simulink library "me375_robot"  (R2023a)
settings: Solver=VariableStepAuto  StartTime=0.0  StopTime=10.0  RelTol=1e-3
libraries: arduinolib x18, simulink x10, arduinosensorlib x2, $bdroot x1
settings Model: Creator=siche  LastModifiedBy=Zamira

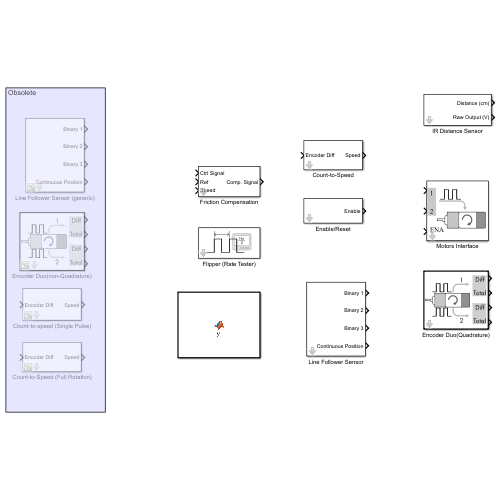
[thumbnail: Simulink's stored preview of the top-level diagram]
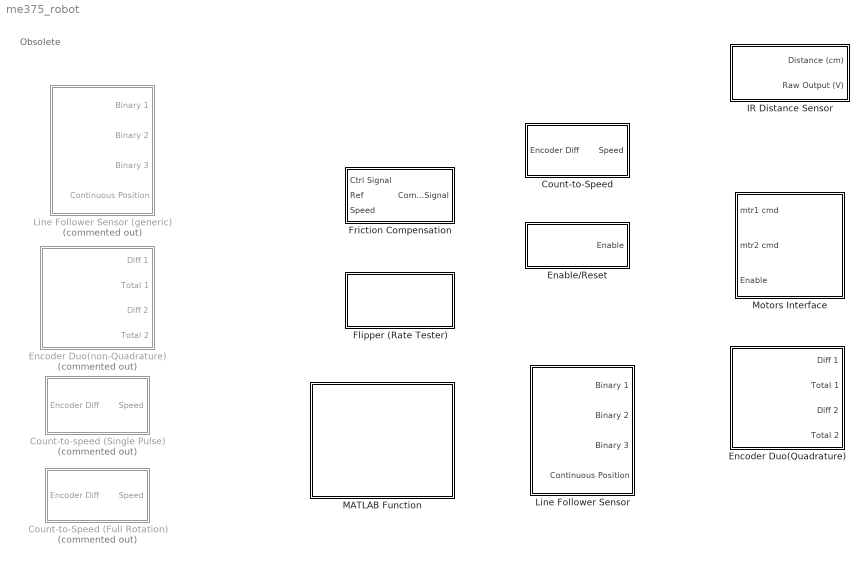
== system me375_robot ==
  note: Obsolete
  Count-to-Speed : Subsystem  mask{cpr=8, Value=184, stop_timeout=15}
      mask prompts: cpr "Window Width"; Value "Count per Wheel Revolution"; stop_timeout "Stop Timeout"
      mask TypeOptions cpr: Pulse Counter/Wrap To Zero/Threshold | Pulse Counter/Constant4/Value | Pulse Counter/Switch/Threshold | Pulse Counter/Switch2/Threshold | Pulse Timing/Constant1/Value
      mask TypeOptions Value: cpr_wheel/Value
      mask TypeOptions stop_timeout: Stop Detection/Wrap To Zero/Threshold | Stop Detection/Switch2/Threshold
      mask DialogControl DescGroupVar Prompt: Encoder Readout Processing
      mask DialogControl DescTextVar Prompt: This block estimates the speed based on the time taken for the encoder to report certain number of counts, specified below as window width. It also accounts for the reduction by the gearbox.
      mask DialogControl Control2 Prompt: This parameter controls the amount of incoming pulses used to estimate the speed. A value too small results in loss in accuracy for high speed, while an overly large value leads to delay at low speeds.
      mask DialogControl Control3 Prompt: The block determines the motor has stopped after recieving this number of consecutive counts of zero.
  Count-to-Speed (Full Rotation) : Subsystem  Commented=on  mask{Value=46, cpr=12, stop_timeout=15}
      mask prompts: Value "Count per Wheel Revolution"; cpr "Count per Rotor Revolution"; stop_timeout "Stop Timeout"
      mask TypeOptions Value: cpr_wheel/Value
      mask TypeOptions cpr: Pulse Counter/Wrap To Zero/Threshold | Pulse Counter/Constant4/Value | Pulse Counter/Switch/Threshold | Pulse Counter/Switch2/Threshold | Pulse Timing/Constant1/Value
      mask TypeOptions stop_timeout: Stop Detection/Wrap To Zero/Threshold | Stop Detection/Switch2/Threshold
      mask DialogControl DescGroupVar Prompt: Encoder Readout Processing
      mask DialogControl DescTextVar Prompt: This block estimates the speed of a motor from the number of encoder pulses recieved since the last iteration of the control loop
      mask DialogControl Control2 Prompt: Encoder count per revolution of the rotor before gearbox. Use 3 for non-quadrature encoder, 12 for quadrature encoder
      mask DialogControl Control3 Prompt: The block determines the motor has stopped after recieving this number of consecutive counts of zero.
  Count-to-speed (Single Pulse) : Subsystem  Commented=on  mask{Value=46, Threshold=15}
      mask prompts: Value "Count per Revolution"; Threshold "Stopping Timeout"
      mask TypeOptions Value: cpr/Value
      mask TypeOptions Threshold: Stop Detection/Wrap To Zero/Threshold
      mask DialogControl DescGroupVar Prompt: Wheel Speed Calculation from Encoder Output
      mask DialogControl DescTextVar Prompt: This block estimates the speed of a motor from the number of encoder pulses recieved since the last iteration of the control loop.
      mask DialogControl Control2 Prompt: Note: This block assumes no more than one incoming encoder count per iteration. If more than one encoder count is expected, one should utilize the Count-to-Speed(Full Rotation) block to avoid exceeding the range of measurement.
      mask DialogControl Control4 Prompt: Count per Revolution = (encoder count per revolution of the motor) x (gear ratio)
      mask DialogControl Control3 Prompt: The block determines the motor has stopped after recieving this number of consecutive counts of zero.
  Enable/Reset : Subsystem  mask{PinEnable=20, enable_override=off}
      mask prompts: PinEnable "Pin number"; enable_override "Button Override"
      mask TypeOptions PinEnable: External Interrupt/Pin
      mask DialogControl DescGroupVar Prompt: Enable/Rest
      mask DialogControl DescTextVar Prompt: Waits for a specified pin to go HIGH before sending out a HIGH as well. This allows one to use external hardware, like a button, to "enable" the connecting block to start functioning.
      mask DialogControl Control2 Prompt: If checked, the robot will start running right after the simulation starts instead of waiting for the button to be pressed.
  Encoder Duo(Quadrature) : Subsystem  TreatAsAtomicUnit=on  mask{mtr_2_dir=on, InputA_enc2=18, InputB_enc2=19, mtr_1_dir=off, InputA_enc1=3, InputB_enc1=2}
      mask prompts: mtr_2_dir "Reverse"; InputA_enc2 "Input A:"; InputB_enc2 "Input B:"; mtr_1_dir "Reverse"; InputA_enc1 "Input A:"; InputB_enc1 "Input B:"
      mask TypeOptions InputA_enc2: Encoder1/InputA
      mask TypeOptions InputB_enc2: Encoder1/InputB
      mask TypeOptions InputA_enc1: Encoder/InputA
      mask TypeOptions InputB_enc1: Encoder/InputB
      mask DialogControl DescTextVar Prompt: Interface with an encoder when only one external interrupt pin is available on the Arduino side. Resolution is 3 counts per revolution of the rotor.
      mask DialogControl ParameterGroupVar Prompt: Pin Settings
      mask DialogControl Container4 Prompt: Motor 1
      mask DialogControl Container5 Prompt: Motor 2
      mask Display: image('encoder_img.svg');
  Encoder Duo(non-Quadrature) : Subsystem  Commented=on  TreatAsAtomicUnit=on  mask{mtr_1_dir=off, pin_intr_1=2, pin_non_intr_1=4, mtr_2_dir=on, pin_intr_2=3, pin_non_intr_2=5, intr_pulledUp_1=on, non_intr_pulledUp_2=Input Pullup, intr_pulledUp_2=on, non_intr_pulledUp_1=Input Pullup, isInputPullup=on}
      mask prompts: mtr_1_dir "Reverse"; pin_intr_1 "Interrupt Pin"; pin_non_intr_1 "Non-interrupt Pin"; mtr_2_dir "Reverse"; pin_intr_2 "Interrupt Pin"; pin_non_intr_2 "Non-interrupt Pin"; intr_pulledUp_1 "Pull-Up Input Pin"; non_intr_pulledUp_2 "Pin mode:"; intr_pulledUp_2 "Pull-Up Input Pin"; non_intr_pulledUp_1 "Pin mode:"; isInputPullup "Pull up"
      mask TypeOptions pin_intr_1: External Interrupt/Pin
      mask TypeOptions pin_non_intr_1:
      | Function-Call
      | Subsystem/Digital Input1/pinNumber
      mask TypeOptions pin_intr_2: External Interrupt1/Pin
      mask TypeOptions pin_non_intr_2:
      | Function-Call
      | Subsystem1/Digital Input1/pinNumber
      mask TypeOptions intr_pulledUp_1: External Interrupt/PullUp
      mask TypeOptions non_intr_pulledUp_2:
      | Function-Call
      | Subsystem1/Digital Input1/mode
      mask TypeOptions intr_pulledUp_2: External Interrupt1/PullUp
      mask TypeOptions non_intr_pulledUp_1:
      | Function-Call
      | Subsystem/Digital Input1/mode
      mask DialogControl DescTextVar Prompt: Interface with an encoder when only one external interrupt pin is available on the Arduino side. Resolution is 3 counts per revolution of the rotor.
      mask DialogControl ParameterGroupVar Prompt: Pin Settings
      mask DialogControl Container4 Prompt: Motor 1
      mask DialogControl Container5 Prompt: Motor 2
      mask DialogControl Container3 Prompt: Pull Up Input
      mask DialogControl Control2 Prompt: The encoders on the Skitter robot require pull-up resistors. Uncheck this box if the resistors are available from the driver board.
      mask Display: image('encoder_img.svg');
  Flipper (Rate Tester) : Subsystem  mask{pinNumber=37}
      mask prompts: pinNumber "Pin number:"
      mask TypeOptions pinNumber: Digital Output/pinNumber
      mask DialogControl DescGroupVar Prompt: Pin State "Flipper"
      mask DialogControl DescTextVar Prompt: For loop rate testing. Use a frequency measurement device (e.g., oscilliscope or multimeter) across the set pin and GND. The frequency at which the control loop runs is twice the measured frequency.
      mask Display: image('flipper_img.svg',[12 8 80 40]);
  Friction Compensation : Subsystem  mask{fric_val=0}
      mask prompts: fric_val "Deadband"
      mask TypeOptions fric_val: Constant1/Value
      mask DialogControl Control2 Prompt: Put the deadband value below to compensate for it:
  IR Distance Sensor : Subsystem  mask{pinNumber=0, CalibValsEnabled=off, Gain4=-4.3019, Gain5=239.1904, Gain6=-0.6848, Gain7=48.1191}
      mask prompts: pinNumber "Pin Number: A"; CalibValsEnabled "Enable Editing"; Gain4 "a1"; Gain5 "k1"; Gain6 "a2"; Gain7 "k2"
      mask TypeOptions pinNumber: Analog Input/pinNumber
      mask TypeOptions Gain4: Gain4/Gain
      mask TypeOptions Gain5: Gain5/Gain
      mask TypeOptions Gain6: Gain6/Gain
      mask TypeOptions Gain7: Gain7/Gain
      mask DialogControl DescTextVar Prompt: This block reads output from a SHARP GP2Y0A21YK0F infrared distance sensor via a 5V/10bit analog input pin.
      mask DialogControl Container4 Prompt: Pin
      mask DialogControl Control2 Prompt: Select analog input pin for the sensor.
      mask DialogControl Container5 Prompt: Calibration
      mask DialogControl Control3 Prompt: The voltage output (u) of the sensor is converted to distance in centimeters (D) by the sum of two exponential functions:
  Line Follower Sensor : Subsystem  mask{Value=650, cont_thresh=256}
      mask prompts: Value "Binary Threshold"; cont_thresh "Continuous Position Correction Threshold"
      mask TypeOptions Value: bin_threshold/Value
      mask TypeOptions cont_thresh: Averaging/Constant/Value | Averaging/Constant1/Value | Averaging/Switch/Threshold | Averaging/Switch1/Threshold
      mask DialogControl Container2 Prompt: Line Follower
      mask DialogControl Control3 Prompt: Uses the three light sensors to determine where the line is likely to be.
      mask DialogControl ParameterGroupVar Prompt: Parameter
      mask DialogControl Control2 Prompt: The Binary Threshold sets the cutoff for the sensors' raw readings, which range from 0 to 1024, before it outputs that it has detected something.
  Line Follower Sensor (generic) : Subsystem  Commented=on  mask{Value=650}
      mask prompts: Value "Binary Threshold"
      mask TypeOptions Value: bin_threshold/Value
      mask DialogControl Container2 Prompt: Line Follower
      mask DialogControl Control3 Prompt: Uses the three light sensors to determine where the line is likely to be.
      mask DialogControl ParameterGroupVar Prompt: Parameter
      mask DialogControl Control2 Prompt: The Binary Threshold sets the cutoff for the sensors' raw readings, which range from 0 to 1024, before it outputs that it has detected something.
  MATLAB Function : MATLAB Function  TreatAsAtomicUnit=on
  Motors Interface : Subsystem  mask{Value=1, pinNumber0=6, pinNumber2=7, pinNumber1=8, pinNumber3=9, desiredFrequency=31372.55}
      mask prompts: Value "u="; pinNumber0 "Out 1"; pinNumber2 "Out 2"; pinNumber1 "Out 1"; pinNumber3 "Out 2"; desiredFrequency "Desired:"
      mask TypeOptions Value: max_input_scaling/Value
      mask TypeOptions pinNumber0: PWM/pinNumber
      mask TypeOptions pinNumber2: PWM2/pinNumber
      mask TypeOptions pinNumber1: PWM1/pinNumber
      mask TypeOptions pinNumber3: PWM3/pinNumber
      mask TypeOptions desiredFrequency: PWM/desiredFrequency | PWM1/desiredFrequency | PWM2/desiredFrequency | PWM3/desiredFrequency
      mask DialogControl DescGroupVar Prompt: PWM Speed Control Interface
      mask DialogControl DescTextVar Prompt: This block converts a control signal to a PWM signal with appropriate duty cycle.
      mask DialogControl Container5 Prompt: Control Signal Range
      mask DialogControl Control2 Prompt: The input control signal should have a value between [-u, u]
      mask DialogControl ParameterGroupVar Prompt: Output Pin Settings
      mask DialogControl Container3 Prompt: Motor 1
      mask DialogControl Container4 Prompt: Motor 2
      mask DialogControl Container7 Prompt: PWM Frequency
      mask Display: image('motor_interface_img.svg');

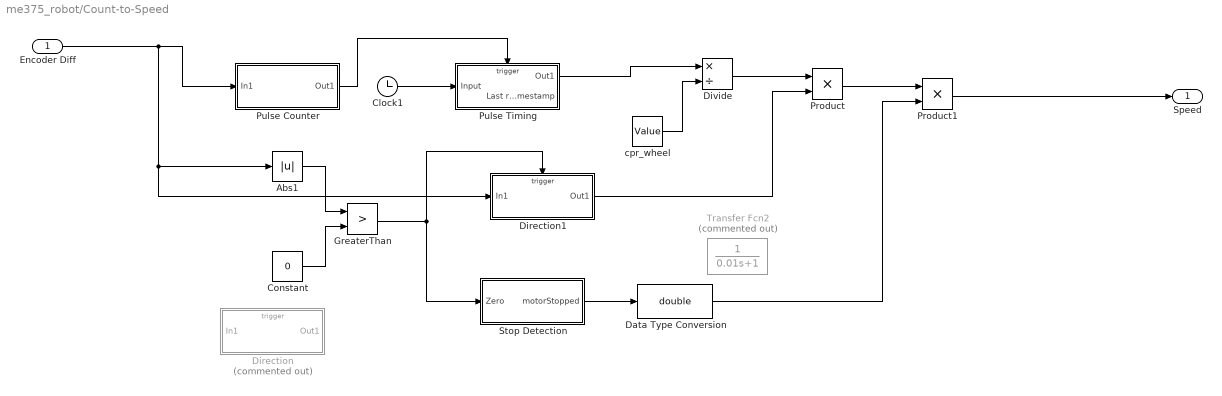
== system me375_robot/Count-to-Speed ==
  Encoder Diff : Inport
  Abs1 : Abs  SaturateOnIntegerOverflow=off
  Clock1 : Clock
  Constant : Constant  Value=0
  Data Type Conversion : DataTypeConversion  OutDataTypeStr=double  SaturateOnIntegerOverflow=off  RndMeth=Floor
  Direction : Subsystem  Commented=on  TreatAsAtomicUnit=on
  Direction1 : Subsystem  TreatAsAtomicUnit=on
  Divide : Product  Inputs=*/
  GreaterThan : RelationalOperator  Operator=>  OutDataTypeStr=boolean  RndMeth=Simplest  InputSameDT=off
  Product : Product
  Product1 : Product
  Pulse Counter : Subsystem
  Pulse Timing : Subsystem  TreatAsAtomicUnit=on
  Stop Detection : Subsystem
  Transfer Fcn2 : TransferFcn  Commented=on  Denominator=[0.01 1]
  cpr_wheel : Constant  Value=Value
  Speed : Outport
  wires:
  Product1/1 -> Speed/1
  cpr_wheel/1 -> Divide/2
  Product/1 -> Product1/1
  Divide/1 -> Product/1
  Abs1/1 -> GreaterThan/1
  Clock1/1 -> Pulse Timing/1(Input)
  Pulse Timing/1(Out1) -> Divide/1
  Constant/1 -> GreaterThan/2
  Pulse Counter/1(Out1) -> Pulse Timing/Trigger
  Encoder Diff/1 -> Pulse Counter/1(In1), Abs1/1, Direction1/1(In1)
  GreaterThan/1 -> Stop Detection/1(Zero), Direction1/Trigger
  Direction1/1(Out1) -> Product/2
  Data Type Conversion/1 -> Product1/2
  Stop Detection/1(motorStopped) -> Data Type Conversion/1

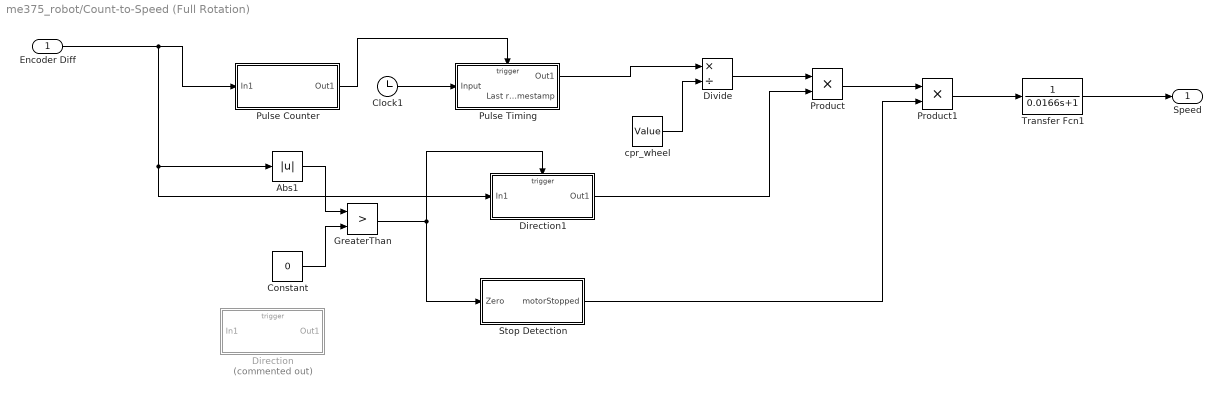
== system me375_robot/Count-to-Speed (Full Rotation) ==
  Encoder Diff : Inport
  Abs1 : Abs  SaturateOnIntegerOverflow=off
  Clock1 : Clock
  Constant : Constant  Value=0
  Direction : Subsystem  Commented=on  TreatAsAtomicUnit=on
  Direction1 : Subsystem  TreatAsAtomicUnit=on
  Divide : Product  Inputs=*/
  GreaterThan : RelationalOperator  Operator=>  OutDataTypeStr=boolean  RndMeth=Simplest  InputSameDT=off
  Product : Product
  Product1 : Product
  Pulse Counter : Subsystem
  Pulse Timing : Subsystem  TreatAsAtomicUnit=on
  Stop Detection : Subsystem
  Transfer Fcn1 : TransferFcn  Denominator=[0.0166 1]
  cpr_wheel : Constant  Value=Value
  Speed : Outport
  wires:
  GreaterThan/1 -> Direction1/Trigger, Stop Detection/1(Zero)
  Encoder Diff/1 -> Direction1/1(In1), Abs1/1, Pulse Counter/1(In1)
  Pulse Counter/1(Out1) -> Pulse Timing/Trigger
  Constant/1 -> GreaterThan/2
  Pulse Timing/1(Out1) -> Divide/1
  Clock1/1 -> Pulse Timing/1(Input)
  Abs1/1 -> GreaterThan/1
  Divide/1 -> Product/1
  Direction1/1(Out1) -> Product/2
  Product/1 -> Product1/1
  Stop Detection/1(motorStopped) -> Product1/2
  cpr_wheel/1 -> Divide/2
  Product1/1 -> Transfer Fcn1/1
  Transfer Fcn1/1 -> Speed/1

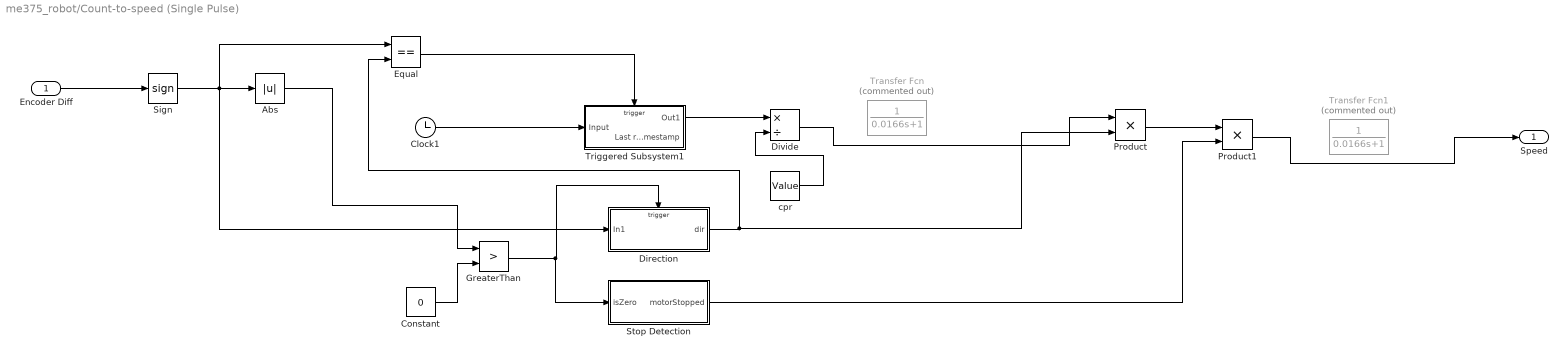
== system me375_robot/Count-to-speed (Single Pulse) ==
  Encoder Diff : Inport
  Abs : Abs  SaturateOnIntegerOverflow=off
  Clock1 : Clock
  Constant : Constant  Value=0
  Direction : Subsystem  TreatAsAtomicUnit=on
  Divide : Product  Inputs=*/
  Equal : RelationalOperator  Operator===  OutDataTypeStr=boolean  RndMeth=Simplest  InputSameDT=off
  GreaterThan : RelationalOperator  Operator=>  OutDataTypeStr=boolean  RndMeth=Simplest  InputSameDT=off
  Product : Product
  Product1 : Product
  Sign : Signum
  Stop Detection : Subsystem
  Transfer Fcn : TransferFcn  Commented=on  Denominator=[0.0166 1]
  Transfer Fcn1 : TransferFcn  Commented=on  Denominator=[0.0166 1]
  Triggered Subsystem1 : Subsystem  TreatAsAtomicUnit=on
  cpr : Constant  Value=Value
  Speed : Outport
  wires:
  GreaterThan/1 -> Stop Detection/1(isZero), Direction/Trigger
  Constant/1 -> GreaterThan/2
  Triggered Subsystem1/1(Out1) -> Divide/1
  Clock1/1 -> Triggered Subsystem1/1(Input)
  Abs/1 -> GreaterThan/1
  Direction/1(dir) -> Product/2, Equal/2
  Product/1 -> Product1/1
  Stop Detection/1(motorStopped) -> Product1/2
  Encoder Diff/1 -> Sign/1
  Sign/1 -> Equal/1, Direction/1(In1), Abs/1
  Equal/1 -> Triggered Subsystem1/Trigger
  cpr/1 -> Divide/2
  Product1/1 -> Speed/1
  Divide/1 -> Product/1

== system me375_robot/Enable//Reset ==
  Constant : Constant  Value=enable_override
  Cool Down : TransferFcn  Denominator=[0.1 1]
  Data Type Conversion : DataTypeConversion  SaturateOnIntegerOverflow=off  RndMeth=Floor
  Data Type Conversion1 : DataTypeConversion  OutDataTypeStr=double  SaturateOnIntegerOverflow=off  RndMeth=Floor
  Digital Input : arduinolib/Digital Input  pinNumber=5  mode=Input Pullup  Direction=input  SampleTime=0.02  blockPlatform=arduino
  External Interrupt : arduinolib/External Interrupt  Pin=PinEnable  PullUp=on  Mode=FALLING  InterruptSimulationInput=off
  OR : Logic  Operator=OR  IconShape=distinctive  AllPortsSameDT=off  OutDataTypeStr=boolean
  RT : RateTransition  Deterministic=off  OutPortSampleTime=0.002
  RT1 : RateTransition  Deterministic=off
  Subsystem : Subsystem
  Enable : Outport
  wires:
  RT/1 -> Data Type Conversion/1
  Subsystem/1(Enable Out) -> RT/1
  RT1/1 -> Subsystem/1(Cool Down Signal)
  Data Type Conversion/1 -> OR/2, Cool Down/1
  Cool Down/1 -> RT1/1
  Constant/1 -> OR/1
  OR/1 -> Data Type Conversion1/1
  Data Type Conversion1/1 -> Enable/1
  Digital Input/1 -> Subsystem/Trigger

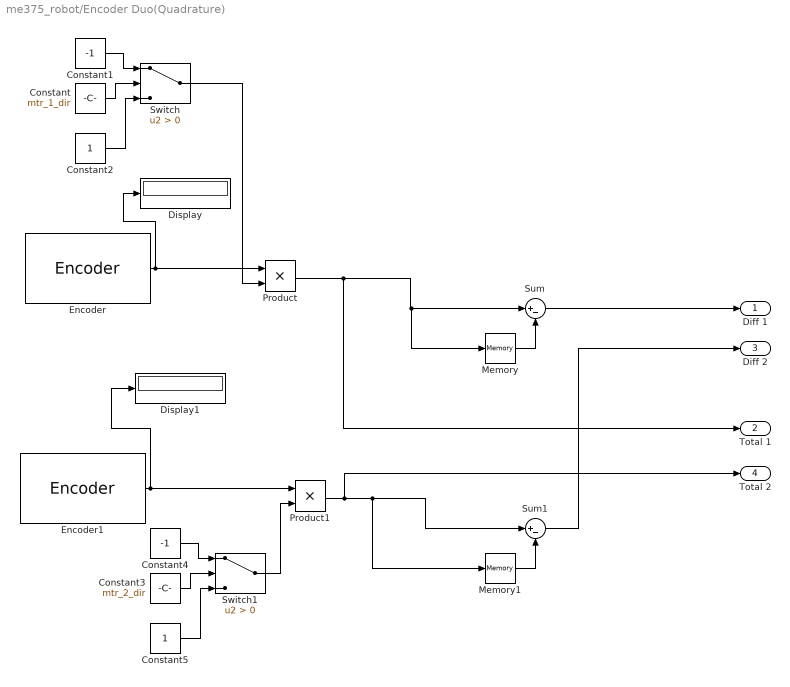
== system me375_robot/Encoder Duo(Quadrature) ==
  Constant : Constant  Value=mtr_1_dir
  Constant1 : Constant  Value=-1
  Constant2 : Constant
  Constant3 : Constant  Value=mtr_2_dir
  Constant4 : Constant  Value=-1
  Constant5 : Constant
  Display : Display
  Display1 : Display
  Encoder : arduinosensorlib/Encoder  InputA=InputA_enc1  InputB=InputB_enc1  Mode=No reset  SampleTime=-1
  Encoder1 : arduinosensorlib/Encoder  InputA=InputA_enc2  InputB=InputB_enc2  Mode=No reset  SampleTime=-1
  Memory : Memory
  Memory1 : Memory
  Product : Product
  Product1 : Product
  Sum : Sum  Inputs=|+-
  Sum1 : Sum  Inputs=|+-
  Switch : Switch  Criteria=u2 > Threshold  SaturateOnIntegerOverflow=off  InputSameDT=off
  Switch1 : Switch  Criteria=u2 > Threshold  SaturateOnIntegerOverflow=off  InputSameDT=off
  Diff 1 : Outport
  Total 1 : Outport  Port=2
  Diff 2 : Outport  Port=3
  Total 2 : Outport  Port=4
  wires:
  Memory/1 -> Sum/2
  Sum/1 -> Diff 1/1
  Sum1/1 -> Diff 2/1
  Memory1/1 -> Sum1/2
  Constant/1 -> Switch/2
  Constant1/1 -> Switch/1
  Constant2/1 -> Switch/3
  Product/1 -> Total 1/1, Memory/1, Sum/1
  Switch/1 -> Product/2
  Constant5/1 -> Switch1/3
  Switch1/1 -> Product1/2
  Constant4/1 -> Switch1/1
  Constant3/1 -> Switch1/2
  Product1/1 -> Total 2/1, Memory1/1, Sum1/1
  Encoder/1 -> Display/1, Product/1
  Encoder1/1 -> Display1/1, Product1/1

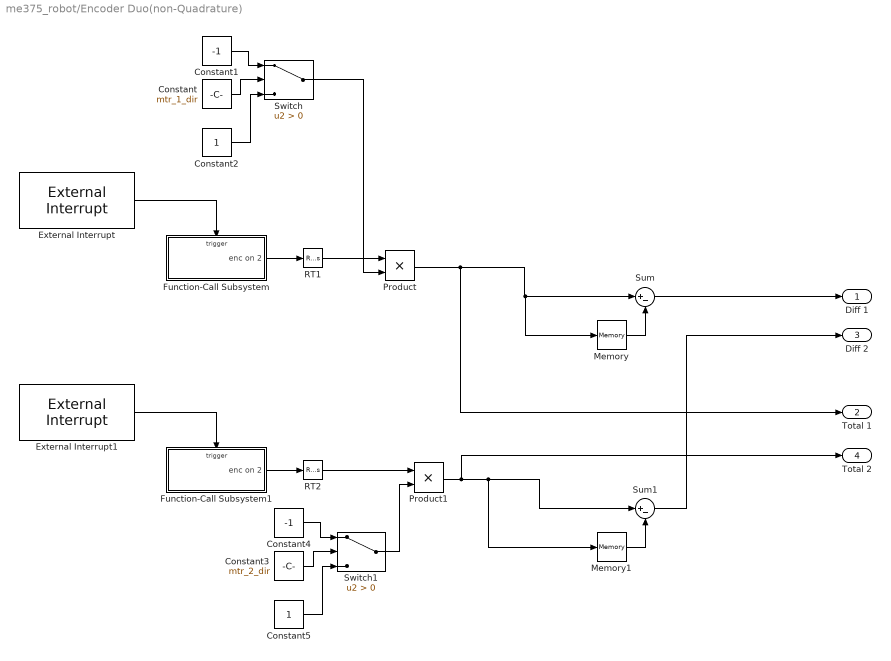
== system me375_robot/Encoder Duo(non-Quadrature) ==
  Constant : Constant  Value=mtr_1_dir
  Constant1 : Constant  Value=-1
  Constant2 : Constant
  Constant3 : Constant  Value=mtr_2_dir
  Constant4 : Constant  Value=-1
  Constant5 : Constant
  External Interrupt : arduinolib/External Interrupt  Pin=pin_intr_1  PullUp=on  Mode=RISING  InterruptSimulationInput=off
  External Interrupt1 : arduinolib/External Interrupt  Pin=pin_intr_2  PullUp=on  Mode=RISING  InterruptSimulationInput=off
  Function-Call Subsystem : Subsystem  TreatAsAtomicUnit=on
  Function-Call Subsystem1 : Subsystem  TreatAsAtomicUnit=on
  Memory : Memory
  Memory1 : Memory
  Product : Product
  Product1 : Product
  RT1 : RateTransition  Deterministic=off  OutPortSampleTime=0.002
  RT2 : RateTransition  Deterministic=off  OutPortSampleTime=0.002
  Sum : Sum  Inputs=|+-
  Sum1 : Sum  Inputs=|+-
  Switch : Switch  Criteria=u2 > Threshold  SaturateOnIntegerOverflow=off  InputSameDT=off
  Switch1 : Switch  Criteria=u2 > Threshold  SaturateOnIntegerOverflow=off  InputSameDT=off
  Diff 1 : Outport
  Total 1 : Outport  Port=2
  Diff 2 : Outport  Port=3
  Total 2 : Outport  Port=4
  wires:
  Function-Call Subsystem/1(enc on 2) -> RT1/1
  Memory/1 -> Sum/2
  External Interrupt/1 -> Function-Call Subsystem/Trigger
  Sum/1 -> Diff 1/1
  Function-Call Subsystem1/1(enc on 2) -> RT2/1
  Sum1/1 -> Diff 2/1
  External Interrupt1/1 -> Function-Call Subsystem1/Trigger
  Memory1/1 -> Sum1/2
  Constant/1 -> Switch/2
  Constant1/1 -> Switch/1
  Constant2/1 -> Switch/3
  RT1/1 -> Product/1
  Product/1 -> Total 1/1, Memory/1, Sum/1
  Switch/1 -> Product/2
  Constant5/1 -> Switch1/3
  Switch1/1 -> Product1/2
  Constant4/1 -> Switch1/1
  Constant3/1 -> Switch1/2
  RT2/1 -> Product1/1
  Product1/1 -> Total 2/1, Memory1/1, Sum1/1

== system me375_robot/Flipper (Rate Tester) ==
  Constant3 : Constant
  Digital Output : arduinolib/Digital Output  pinNumber=pinNumber  Direction=output  blockPlatform=arduino
  Memory1 : Memory
  XOR : Logic  Operator=XOR  IconShape=distinctive  AllPortsSameDT=off  OutDataTypeStr=boolean
  wires:
  Constant3/1 -> XOR/2
  Memory1/1 -> XOR/1
  XOR/1 -> Memory1/1, Digital Output/1

== system me375_robot/Friction Compensation ==
  Ctrl Signal : Inport
  Ref : Inport  Port=2
  Speed : Inport  Port=3
  AND : Logic  Operator=OR  IconShape=distinctive  AllPortsSameDT=off  OutDataTypeStr=boolean
  Constant : Constant  Value=0
  Constant1 : Constant  Value=fric_val
  Equal : RelationalOperator  Operator===  OutDataTypeStr=boolean  RndMeth=Simplest  InputSameDT=off
  NotEqual : RelationalOperator  Operator=~=  OutDataTypeStr=boolean  RndMeth=Simplest  InputSameDT=off
  Product : Product
  Sign : Signum
  Sum : Sum  Inputs=|++
  Switch : Switch  Criteria=u2 > Threshold  SaturateOnIntegerOverflow=off  InputSameDT=off
  Comp. Signal : Outport
  wires:
  Ref/1 -> Sign/1, NotEqual/1
  Switch/1 -> Sum/2
  Sum/1 -> Comp. Signal/1
  Product/1 -> Switch/1
  AND/1 -> Switch/2
  Sign/1 -> Product/1
  Equal/1 -> AND/2
  NotEqual/1 -> AND/1
  Speed/1 -> Equal/2
  Constant1/1 -> Product/2
  Ctrl Signal/1 -> Sum/1
  Constant/1 -> NotEqual/2, Switch/3, Equal/1

== system me375_robot/IR Distance Sensor ==
  Analog Input : arduinolib/Analog Input  pinNumber=pinNumber  ReadResultsOnly=off  ConversionTriggerSource=Software  ExternalTriggerType=uint32( 0 )  OutputDataType=uint16  EnableConversionCompleteNotify=off  EnableOuputStatus=off  SampleTime=-1  blockPlatform=arduino
  Data Type Conversion2 : DataTypeConversion  OutDataTypeStr=double  SaturateOnIntegerOverflow=off  RndMeth=Floor
  Gain2 : Gain  Gain=5/1023
  Gain4 : Gain  Gain=Gain4
  Gain5 : Gain  Gain=Gain5
  Gain6 : Gain  Gain=Gain6
  Gain7 : Gain  Gain=Gain7
  Math Function : Math
  Math Function1 : Math
  Sum1 : Sum  Inputs=|++
  Transfer Fcn : TransferFcn  Denominator=[0.0166 1]
  Distance (cm) : Outport
  Raw Output (V) : Outport  Port=2
  wires:
  Math Function1/1 -> Gain7/1
  Gain6/1 -> Math Function1/1
  Analog Input/1 -> Gain2/1
  Gain2/1 -> Raw Output (V)/1, Data Type Conversion2/1
  Gain7/1 -> Sum1/2
  Gain4/1 -> Math Function/1
  Gain5/1 -> Sum1/1
  Math Function/1 -> Gain5/1
  Data Type Conversion2/1 -> Gain6/1, Gain4/1
  Sum1/1 -> Transfer Fcn/1
  Transfer Fcn/1 -> Distance (cm)/1

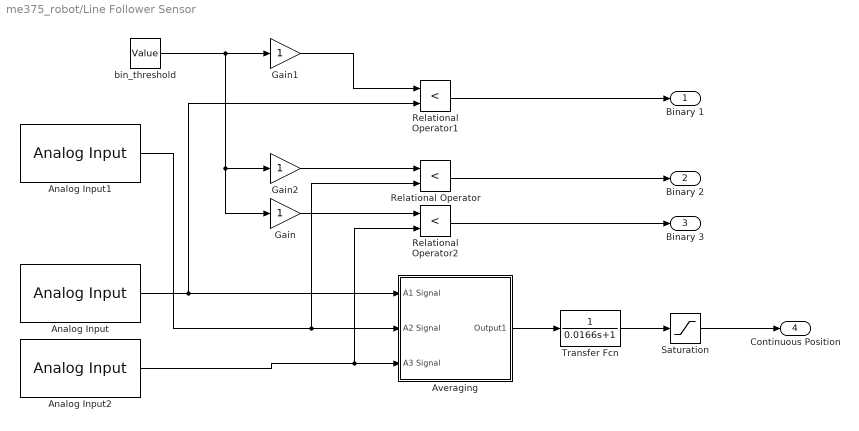
== system me375_robot/Line Follower Sensor ==
  Analog Input : arduinolib/Analog Input  pinNumber=1  ReadResultsOnly=off  ConversionTriggerSource=Software  ExternalTriggerType=uint32( 0 )  OutputDataType=uint16  EnableConversionCompleteNotify=off  EnableOuputStatus=off  SampleTime=-1  blockPlatform=arduino
  Analog Input1 : arduinolib/Analog Input  pinNumber=2  ReadResultsOnly=off  ConversionTriggerSource=Software  ExternalTriggerType=uint32( 0 )  OutputDataType=uint16  EnableConversionCompleteNotify=off  EnableOuputStatus=off  SampleTime=-1  blockPlatform=arduino
  Analog Input2 : arduinolib/Analog Input  pinNumber=3  ReadResultsOnly=off  ConversionTriggerSource=Software  ExternalTriggerType=uint32( 0 )  OutputDataType=uint16  EnableConversionCompleteNotify=off  EnableOuputStatus=off  SampleTime=-1  blockPlatform=arduino
  Averaging : Subsystem
  Gain : Gain
  Gain1 : Gain
  Gain2 : Gain
  Relational Operator : RelationalOperator  Operator=<  OutDataTypeStr=boolean  RndMeth=Simplest  InputSameDT=off
  Relational Operator1 : RelationalOperator  Operator=<  OutDataTypeStr=boolean  RndMeth=Simplest  InputSameDT=off
  Relational Operator2 : RelationalOperator  Operator=<  OutDataTypeStr=boolean  RndMeth=Simplest  InputSameDT=off
  Saturation : Saturate  UpperLimit=1  LowerLimit=-1
  Transfer Fcn : TransferFcn  Denominator=[0.0166 1]
  bin_threshold : Constant  Value=Value
  Binary 1 : Outport
  Binary 2 : Outport  Port=2
  Binary 3 : Outport  Port=3
  Continuous Position : Outport  Port=4
  wires:
  Analog Input/1 -> Relational Operator1/2, Averaging/1(A1 Signal)
  Averaging/1(Output1) -> Transfer Fcn/1
  Transfer Fcn/1 -> Saturation/1
  Saturation/1 -> Continuous Position/1
  Analog Input2/1 -> Relational Operator2/2, Averaging/3(A3 Signal)
  Gain/1 -> Relational Operator2/1
  Gain1/1 -> Relational Operator1/1
  Gain2/1 -> Relational Operator/1
  Relational Operator2/1 -> Binary 3/1
  Relational Operator1/1 -> Binary 1/1
  Analog Input1/1 -> Relational Operator/2, Averaging/2(A2 Signal)
  Relational Operator/1 -> Binary 2/1
  bin_threshold/1 -> Gain2/1, Gain/1, Gain1/1

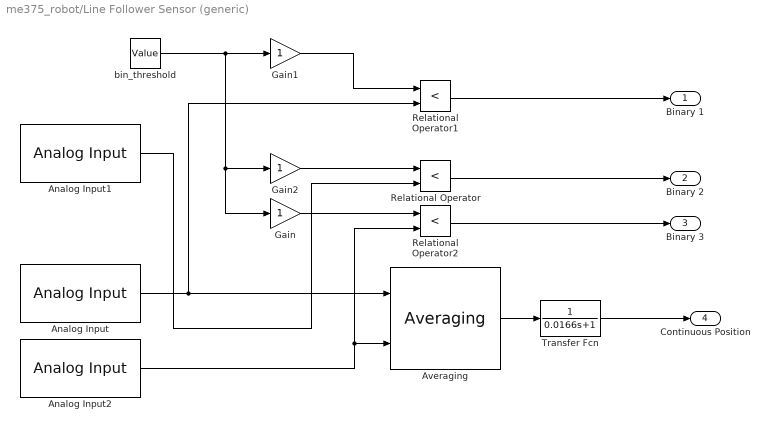
== system me375_robot/Line Follower Sensor (generic) ==
  Analog Input : arduinolib/Analog Input  pinNumber=1  ReadResultsOnly=off  ConversionTriggerSource=Software  ExternalTriggerType=uint32( 0 )  OutputDataType=uint16  EnableConversionCompleteNotify=off  EnableOuputStatus=off  SampleTime=-1  blockPlatform=arduino
  Analog Input1 : arduinolib/Analog Input  pinNumber=2  ReadResultsOnly=off  ConversionTriggerSource=Software  ExternalTriggerType=uint32( 0 )  OutputDataType=uint16  EnableConversionCompleteNotify=off  EnableOuputStatus=off  SampleTime=-1  blockPlatform=arduino
  Analog Input2 : arduinolib/Analog Input  pinNumber=3  ReadResultsOnly=off  ConversionTriggerSource=Software  ExternalTriggerType=uint32( 0 )  OutputDataType=uint16  EnableConversionCompleteNotify=off  EnableOuputStatus=off  SampleTime=-1  blockPlatform=arduino
  Averaging : $bdroot/Light Sensor (Generic)/Averaging  SystemSampleTime=-1  VariantActivationTime=update diagram  Latency=0  AutoFrameSizeCalculation=off
  Gain : Gain
  Gain1 : Gain
  Gain2 : Gain
  Relational Operator : RelationalOperator  Operator=<  OutDataTypeStr=boolean  RndMeth=Simplest  InputSameDT=off
  Relational Operator1 : RelationalOperator  Operator=<  OutDataTypeStr=boolean  RndMeth=Simplest  InputSameDT=off
  Relational Operator2 : RelationalOperator  Operator=<  OutDataTypeStr=boolean  RndMeth=Simplest  InputSameDT=off
  Transfer Fcn : TransferFcn  Denominator=[0.0166 1]
  bin_threshold : Constant  Value=Value
  Binary 1 : Outport
  Binary 2 : Outport  Port=2
  Binary 3 : Outport  Port=3
  Continuous Position : Outport  Port=4
  wires:
  Analog Input/1 -> Averaging/1, Relational Operator1/2
  Analog Input2/1 -> Averaging/2, Relational Operator2/2
  Gain/1 -> Relational Operator2/1
  Gain1/1 -> Relational Operator1/1
  Gain2/1 -> Relational Operator/1
  Relational Operator2/1 -> Binary 3/1
  Relational Operator1/1 -> Binary 1/1
  Analog Input1/1 -> Relational Operator/2
  Relational Operator/1 -> Binary 2/1
  bin_threshold/1 -> Gain2/1, Gain/1, Gain1/1
  Averaging/1 -> Transfer Fcn/1
  Transfer Fcn/1 -> Continuous Position/1

== system me375_robot/Motors Interface ==
  note: This block maps a speed input from -1 to 1 to PWM output between 0 and 255, and set pin states for direction
  mtr1 cmd : Inport
  mtr2 cmd : Inport  Port=2
  Enable : Inport  Port=3
  Ctrl to Mtr Cmd (Braking) : Subsystem
  Ctrl to Mtr Cmd (Braking)1 : Subsystem
  Divide : Product  Inputs=*/
  Divide1 : Product  Inputs=*/
  PWM : arduinolib/PWM  pinNumber=pinNumber0  frequencyType=Specify  desiredFrequency=desiredFrequency  achievableFrequency=490.2
  PWM1 : arduinolib/PWM  pinNumber=pinNumber1  frequencyType=Specify  desiredFrequency=desiredFrequency  achievableFrequency=490.2
  PWM2 : arduinolib/PWM  pinNumber=pinNumber2  frequencyType=Specify  desiredFrequency=desiredFrequency  achievableFrequency=490.2
  PWM3 : arduinolib/PWM  pinNumber=pinNumber3  frequencyType=Specify  desiredFrequency=desiredFrequency  achievableFrequency=490.2
  Product : Product
  Product1 : Product
  max_input_scaling : Constant  Value=Value
  wires:
  Ctrl to Mtr Cmd (Braking)/1(PWM Out 1) -> PWM2/1
  Ctrl to Mtr Cmd (Braking)/2(PWM Out 2) -> PWM/1
  Ctrl to Mtr Cmd (Braking)1/2(PWM Out 2) -> PWM3/1
  Ctrl to Mtr Cmd (Braking)1/1(PWM Out 1) -> PWM1/1
  mtr2 cmd/1 -> Product1/2
  mtr1 cmd/1 -> Product/2
  Enable/1 -> Product1/1, Product/1
  Product/1 -> Divide/1
  Divide/1 -> Ctrl to Mtr Cmd (Braking)/1(Ctrl Signal in)
  max_input_scaling/1 -> Divide1/2, Divide/2
  Divide1/1 -> Ctrl to Mtr Cmd (Braking)1/1(Ctrl Signal in)
  Product1/1 -> Divide1/1

== system me375_robot/Count-to-Speed/Direction ==
  In1 : Inport
  Trigger : TriggerPort  VariantControl=(inherit)
  Add : Sum
  Add1 : Sum
  Add2 : Sum
  Constant : Constant
  Constant1 : Constant  Value=-1
  Delay : Delay  DelayLength=3
  Delay1 : Delay
  Delay2 : Delay  DelayLength=1
  Switch : Switch  Criteria=u2 > Threshold  SaturateOnIntegerOverflow=off  InputSameDT=off
  Out1 : Outport
  wires:
  Constant1/1 -> Switch/3
  Constant/1 -> Switch/1
  Switch/1 -> Out1/1
  Add2/1 -> Switch/2
  Add/1 -> Add2/2
  Add1/1 -> Add2/1
  Delay/1 -> Add1/1
  Delay1/1 -> Add1/2
  Delay2/1 -> Add/2
  In1/1 -> Delay/1, Delay1/1, Delay2/1, Add/1

== system me375_robot/Count-to-Speed/Direction1 ==
  In1 : Inport
  Trigger : TriggerPort  VariantControl=(inherit)
  Sign : Signum
  Out1 : Outport
  wires:
  In1/1 -> Sign/1
  Sign/1 -> Out1/1

== system me375_robot/Count-to-Speed/Pulse Counter ==
  In1 : Inport
  AND : Logic  Operator=NAND  IconShape=distinctive  AllPortsSameDT=off  OutDataTypeStr=boolean
  Abs : Abs  SaturateOnIntegerOverflow=off
  Constant : Constant  Value=0
  Constant1 : Constant
  Constant4 : Constant  Value=cpr
  Constant5 : Constant  Value=cpr-1
  Memory : Memory
  Sum : Sum  Inputs=|++
  Sum1 : Sum  Inputs=|-+
  Switch : Switch  Threshold=cpr  SaturateOnIntegerOverflow=off  InputSameDT=off
  Switch2 : Switch  Criteria=u2 > Threshold  Threshold=cpr  SaturateOnIntegerOverflow=off  InputSameDT=off
  Switch3 : Switch  Criteria=u2 > Threshold  Threshold=cpr-1  SaturateOnIntegerOverflow=off  InputSameDT=off
  Wrap To Zero : simulink/Discontinuities/Wrap To Zero  Threshold=cpr
  Out1 : Outport
  wires:
  Switch3/1 -> Switch2/1
  Constant5/1 -> Switch3/1
  Sum1/1 -> Switch3/2, Switch3/3
  Switch2/1 -> Memory/1
  Sum/1 -> Wrap To Zero/1, Sum1/2, Switch2/2, Switch2/3
  Constant4/1 -> Sum1/1
  Abs/1 -> Sum/1
  AND/1 -> Out1/1
  Switch/1 -> AND/2
  Constant1/1 -> Switch/3
  Constant/1 -> Switch/1
  Wrap To Zero/1 -> AND/1
  Memory/1 -> Sum/2, Switch/2
  In1/1 -> Abs/1

== system me375_robot/Count-to-Speed/Pulse Timing ==
  Input : Inport
  Trigger : TriggerPort  VariantControl=(inherit)
  Constant1 : Constant  Value=cpr
  Delay : Delay
  Delay1 : Delay  DelayLength=1
  Divide : Product  Inputs=*/
  Gain : Gain  Gain=1/3
  Minus : Sum  Inputs=+-
  Sum : Sum  Inputs=+++
  Unit Delay : UnitDelay  SampleTime=-1  HasFrameUpgradeWarning=on
  Out1 : Outport  InitialOutput=0
  Last round timestamp : Outport  Port=2
  wires:
  Gain/1 -> Out1/1
  Sum/1 -> Gain/1
  Delay1/1 -> Sum/3
  Delay/1 -> Sum/1
  Unit Delay/1 -> Minus/2, Last round timestamp/1
  Divide/1 -> Delay1/1, Delay/1, Sum/2
  Constant1/1 -> Divide/1
  Minus/1 -> Divide/2
  Input/1 -> Minus/1, Unit Delay/1

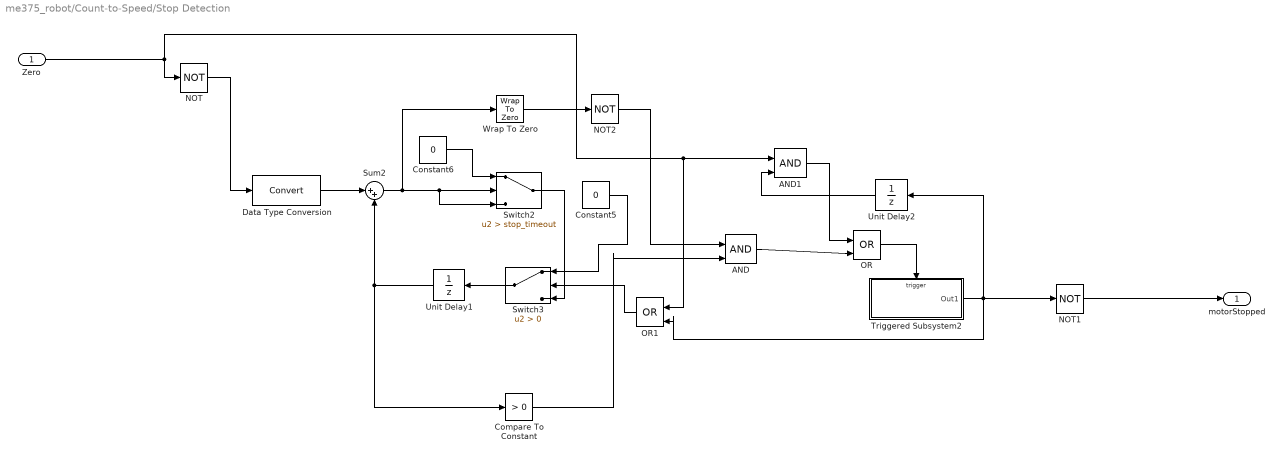
== system me375_robot/Count-to-Speed/Stop Detection ==
  Zero : Inport
  AND : Logic  IconShape=distinctive  AllPortsSameDT=off  OutDataTypeStr=boolean
  AND1 : Logic  IconShape=distinctive  AllPortsSameDT=off  OutDataTypeStr=boolean
  Compare To Constant : simulink/Logic and Bit Operations/Compare To Constant  relop=>  const=0  OutDataTypeStr=boolean
  Constant5 : Constant  Value=0
  Constant6 : Constant  Value=0
  Data Type Conversion : DataTypeConversion  SaturateOnIntegerOverflow=off  RndMeth=Floor
  NOT : Logic  Operator=NOT  IconShape=distinctive  AllPortsSameDT=off  OutDataTypeStr=boolean
  NOT1 : Logic  Operator=NOT  IconShape=distinctive  AllPortsSameDT=off  OutDataTypeStr=boolean
  NOT2 : Logic  Operator=NOT  IconShape=distinctive  AllPortsSameDT=off  OutDataTypeStr=boolean
  OR : Logic  Operator=OR  IconShape=distinctive  AllPortsSameDT=off  OutDataTypeStr=boolean
  OR1 : Logic  Operator=OR  IconShape=distinctive  AllPortsSameDT=off  OutDataTypeStr=boolean
  Sum2 : Sum  Inputs=|++
  Switch2 : Switch  Criteria=u2 > Threshold  Threshold=stop_timeout  SaturateOnIntegerOverflow=off  InputSameDT=off
  Switch3 : Switch  Criteria=u2 > Threshold  SaturateOnIntegerOverflow=off  InputSameDT=off
  Triggered Subsystem2 : Subsystem  TreatAsAtomicUnit=on
  Unit Delay1 : UnitDelay  SampleTime=-1  HasFrameUpgradeWarning=on
  Unit Delay2 : UnitDelay  SampleTime=-1  HasFrameUpgradeWarning=on
  Wrap To Zero : simulink/Discontinuities/Wrap To Zero  Threshold=stop_timeout
  motorStopped : Outport
  wires:
  Unit Delay1/1 -> Compare To Constant/1, Sum2/2
  Zero/1 -> NOT/1, AND1/1, OR1/1
  Switch2/1 -> Switch3/3
  AND1/1 -> OR/1
  Sum2/1 -> Switch2/3, Switch2/2, Wrap To Zero/1
  Data Type Conversion/1 -> Sum2/1
  Switch3/1 -> Unit Delay1/1
  OR1/1 -> Switch3/2
  Triggered Subsystem2/1(Out1) -> OR1/2, NOT1/1, Unit Delay2/1
  NOT/1 -> Data Type Conversion/1
  Unit Delay2/1 -> AND1/2
  Constant6/1 -> Switch2/1
  Constant5/1 -> Switch3/1
  OR/1 -> Triggered Subsystem2/Trigger
  AND/1 -> OR/2
  NOT2/1 -> AND/1
  NOT1/1 -> motorStopped/1
  Compare To Constant/1 -> AND/2
  Wrap To Zero/1 -> NOT2/1

== system me375_robot/Count-to-Speed (Full Rotation)/Direction ==
  In1 : Inport
  Trigger : TriggerPort  VariantControl=(inherit)
  Add : Sum
  Add1 : Sum
  Add2 : Sum
  Constant : Constant
  Constant1 : Constant  Value=-1
  Delay : Delay  DelayLength=3
  Delay1 : Delay
  Delay2 : Delay  DelayLength=1
  Switch : Switch  Criteria=u2 > Threshold  SaturateOnIntegerOverflow=off  InputSameDT=off
  Out1 : Outport
  wires:
  In1/1 -> Add/1, Delay2/1, Delay1/1, Delay/1
  Delay2/1 -> Add/2
  Delay1/1 -> Add1/2
  Delay/1 -> Add1/1
  Add1/1 -> Add2/1
  Add/1 -> Add2/2
  Add2/1 -> Switch/2
  Switch/1 -> Out1/1
  Constant/1 -> Switch/1
  Constant1/1 -> Switch/3

== system me375_robot/Count-to-Speed (Full Rotation)/Direction1 ==
  In1 : Inport
  Trigger : TriggerPort  VariantControl=(inherit)
  Sign : Signum
  Out1 : Outport
  wires:
  Sign/1 -> Out1/1
  In1/1 -> Sign/1

== system me375_robot/Count-to-Speed (Full Rotation)/Pulse Counter ==
  In1 : Inport
  AND : Logic  Operator=NAND  IconShape=distinctive  AllPortsSameDT=off  OutDataTypeStr=boolean
  Abs : Abs  SaturateOnIntegerOverflow=off
  Constant : Constant  Value=0
  Constant1 : Constant
  Constant4 : Constant  Value=cpr
  Constant5 : Constant  Value=cpr-1
  Memory : Memory
  Sum : Sum  Inputs=|++
  Sum1 : Sum  Inputs=|-+
  Switch : Switch  Threshold=cpr  SaturateOnIntegerOverflow=off  InputSameDT=off
  Switch2 : Switch  Criteria=u2 > Threshold  Threshold=cpr  SaturateOnIntegerOverflow=off  InputSameDT=off
  Switch3 : Switch  Criteria=u2 > Threshold  Threshold=cpr-1  SaturateOnIntegerOverflow=off  InputSameDT=off
  Wrap To Zero : simulink/Discontinuities/Wrap To Zero  Threshold=cpr
  Out1 : Outport
  wires:
  In1/1 -> Abs/1
  Memory/1 -> Switch/2, Sum/2
  Wrap To Zero/1 -> AND/1
  Constant/1 -> Switch/1
  Constant1/1 -> Switch/3
  Switch/1 -> AND/2
  AND/1 -> Out1/1
  Abs/1 -> Sum/1
  Constant4/1 -> Sum1/1
  Sum/1 -> Switch2/3, Switch2/2, Sum1/2, Wrap To Zero/1
  Switch2/1 -> Memory/1
  Sum1/1 -> Switch3/3, Switch3/2
  Constant5/1 -> Switch3/1
  Switch3/1 -> Switch2/1

== system me375_robot/Count-to-Speed (Full Rotation)/Pulse Timing ==
  Input : Inport
  Trigger : TriggerPort  VariantControl=(inherit)
  Constant1 : Constant  Value=cpr
  Delay : Delay
  Delay1 : Delay  DelayLength=1
  Divide : Product  Inputs=*/
  Gain : Gain  Gain=1/3
  Minus : Sum  Inputs=+-
  Sum : Sum  Inputs=+++
  Unit Delay : UnitDelay  SampleTime=-1  HasFrameUpgradeWarning=on
  Out1 : Outport  InitialOutput=0
  Last round timestamp : Outport  Port=2
  wires:
  Input/1 -> Unit Delay/1, Minus/1
  Minus/1 -> Divide/2
  Constant1/1 -> Divide/1
  Divide/1 -> Sum/2, Delay/1, Delay1/1
  Unit Delay/1 -> Last round timestamp/1, Minus/2
  Delay/1 -> Sum/1
  Delay1/1 -> Sum/3
  Sum/1 -> Gain/1
  Gain/1 -> Out1/1

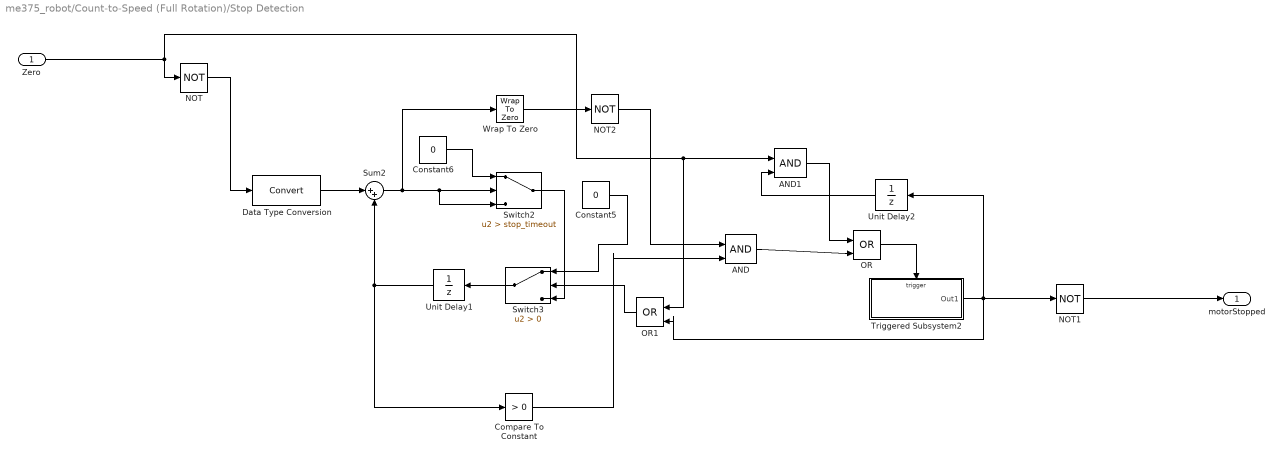
== system me375_robot/Count-to-Speed (Full Rotation)/Stop Detection ==
  Zero : Inport
  AND : Logic  IconShape=distinctive  AllPortsSameDT=off  OutDataTypeStr=boolean
  AND1 : Logic  IconShape=distinctive  AllPortsSameDT=off  OutDataTypeStr=boolean
  Compare To Constant : simulink/Logic and Bit Operations/Compare To Constant  relop=>  const=0  OutDataTypeStr=boolean
  Constant5 : Constant  Value=0
  Constant6 : Constant  Value=0
  Data Type Conversion : DataTypeConversion  SaturateOnIntegerOverflow=off  RndMeth=Floor
  NOT : Logic  Operator=NOT  IconShape=distinctive  AllPortsSameDT=off  OutDataTypeStr=boolean
  NOT1 : Logic  Operator=NOT  IconShape=distinctive  AllPortsSameDT=off  OutDataTypeStr=boolean
  NOT2 : Logic  Operator=NOT  IconShape=distinctive  AllPortsSameDT=off  OutDataTypeStr=boolean
  OR : Logic  Operator=OR  IconShape=distinctive  AllPortsSameDT=off  OutDataTypeStr=boolean
  OR1 : Logic  Operator=OR  IconShape=distinctive  AllPortsSameDT=off  OutDataTypeStr=boolean
  Sum2 : Sum  Inputs=|++
  Switch2 : Switch  Criteria=u2 > Threshold  Threshold=stop_timeout  SaturateOnIntegerOverflow=off  InputSameDT=off
  Switch3 : Switch  Criteria=u2 > Threshold  SaturateOnIntegerOverflow=off  InputSameDT=off
  Triggered Subsystem2 : Subsystem  TreatAsAtomicUnit=on
  Unit Delay1 : UnitDelay  SampleTime=-1  HasFrameUpgradeWarning=on
  Unit Delay2 : UnitDelay  SampleTime=-1  HasFrameUpgradeWarning=on
  Wrap To Zero : simulink/Discontinuities/Wrap To Zero  Threshold=stop_timeout
  motorStopped : Outport
  wires:
  Wrap To Zero/1 -> NOT2/1
  Compare To Constant/1 -> AND/2
  NOT1/1 -> motorStopped/1
  NOT2/1 -> AND/1
  AND/1 -> OR/2
  OR/1 -> Triggered Subsystem2/Trigger
  Constant5/1 -> Switch3/1
  Constant6/1 -> Switch2/1
  Unit Delay2/1 -> AND1/2
  NOT/1 -> Data Type Conversion/1
  Triggered Subsystem2/1(Out1) -> Unit Delay2/1, NOT1/1, OR1/2
  OR1/1 -> Switch3/2
  Switch3/1 -> Unit Delay1/1
  Data Type Conversion/1 -> Sum2/1
  Sum2/1 -> Wrap To Zero/1, Switch2/2, Switch2/3
  AND1/1 -> OR/1
  Switch2/1 -> Switch3/3
  Zero/1 -> OR1/1, AND1/1, NOT/1
  Unit Delay1/1 -> Sum2/2, Compare To Constant/1

== system me375_robot/Count-to-speed (Single Pulse)/Direction ==
  In1 : Inport
  Trigger : TriggerPort  VariantControl=(inherit)
  Add{,1..3} (4 alike) : Sum
  Constant : Constant
  Constant1 : Constant  Value=-1
  Delay : Delay  DelayLength=3
  Delay1 : Delay
  Delay2 : Delay  DelayLength=1
  Delay3 : Delay  DelayLength=4
  Switch : Switch  Criteria=u2 > Threshold  SaturateOnIntegerOverflow=off  InputSameDT=off
  dir : Outport
  wires:
  In1/1 -> Add/1, Delay2/1, Delay1/1, Delay3/1, Delay/1
  Delay2/1 -> Add/2
  Delay1/1 -> Add1/2
  Delay/1 -> Add1/1
  Add1/1 -> Add2/1
  Add/1 -> Add2/2
  Switch/1 -> dir/1
  Constant/1 -> Switch/1
  Constant1/1 -> Switch/3
  Add2/1 -> Add3/2
  Add3/1 -> Switch/2
  Delay3/1 -> Add3/1

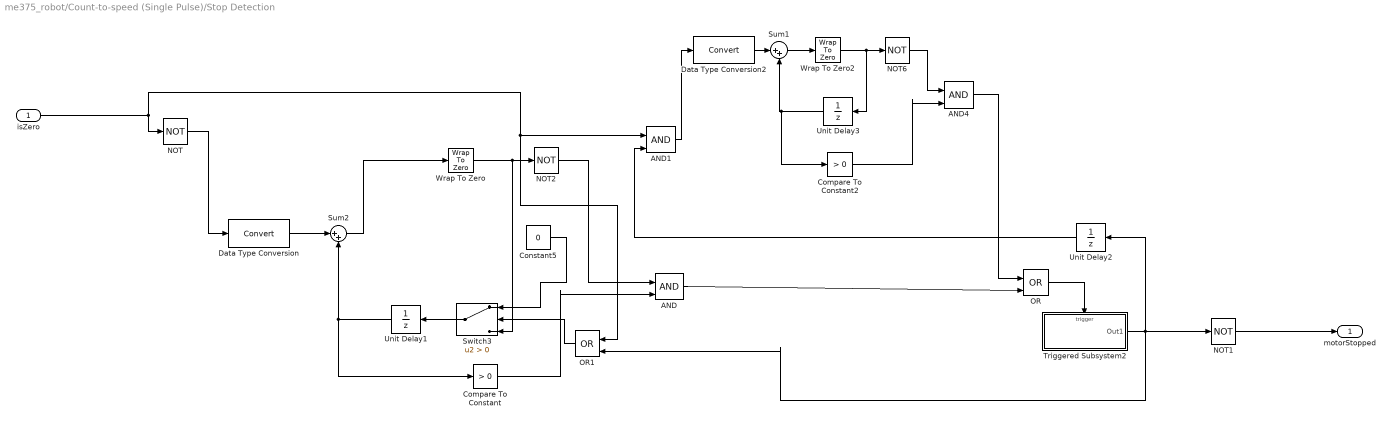
== system me375_robot/Count-to-speed (Single Pulse)/Stop Detection ==
  isZero : Inport
  AND : Logic  IconShape=distinctive  AllPortsSameDT=off  OutDataTypeStr=boolean
  AND1 : Logic  IconShape=distinctive  AllPortsSameDT=off  OutDataTypeStr=boolean
  AND4 : Logic  IconShape=distinctive  AllPortsSameDT=off  OutDataTypeStr=boolean
  Compare To Constant : simulink/Logic and Bit Operations/Compare To Constant  relop=>  const=0  OutDataTypeStr=boolean
  Compare To Constant2 : simulink/Logic and Bit Operations/Compare To Constant  relop=>  const=0  OutDataTypeStr=boolean
  Constant5 : Constant  Value=0
  Data Type Conversion : DataTypeConversion  SaturateOnIntegerOverflow=off  RndMeth=Floor
  Data Type Conversion2 : DataTypeConversion  SaturateOnIntegerOverflow=off  RndMeth=Floor
  NOT{,1..2,6} (4 alike) : Logic  Operator=NOT  IconShape=distinctive  AllPortsSameDT=off  OutDataTypeStr=boolean
  OR : Logic  Operator=OR  IconShape=distinctive  AllPortsSameDT=off  OutDataTypeStr=boolean
  OR1 : Logic  Operator=OR  IconShape=distinctive  AllPortsSameDT=off  OutDataTypeStr=boolean
  Sum1 : Sum  Inputs=|++
  Sum2 : Sum  Inputs=|++
  Switch3 : Switch  Criteria=u2 > Threshold  SaturateOnIntegerOverflow=off  InputSameDT=off
  Triggered Subsystem2 : Subsystem  TreatAsAtomicUnit=on
  Unit Delay1 : UnitDelay  SampleTime=-1  HasFrameUpgradeWarning=on
  Unit Delay2 : UnitDelay  SampleTime=-1  HasFrameUpgradeWarning=on
  Unit Delay3 : UnitDelay  SampleTime=-1  HasFrameUpgradeWarning=on
  Wrap To Zero : simulink/Discontinuities/Wrap To Zero  Threshold=Threshold
  Wrap To Zero2 : simulink/Discontinuities/Wrap To Zero  Threshold=1
  motorStopped : Outport
  wires:
  Compare To Constant/1 -> AND/2
  NOT1/1 -> motorStopped/1
  NOT2/1 -> AND/1
  AND/1 -> OR/2
  OR/1 -> Triggered Subsystem2/Trigger
  Constant5/1 -> Switch3/1
  Unit Delay2/1 -> AND1/2
  NOT/1 -> Data Type Conversion/1
  Triggered Subsystem2/1(Out1) -> Unit Delay2/1, NOT1/1, OR1/2
  OR1/1 -> Switch3/2
  Switch3/1 -> Unit Delay1/1
  Data Type Conversion/1 -> Sum2/1
  Sum2/1 -> Wrap To Zero/1
  Wrap To Zero/1 -> Switch3/3, NOT2/1
  Unit Delay1/1 -> Sum2/2, Compare To Constant/1
  isZero/1 -> OR1/1, AND1/1, NOT/1
  Sum1/1 -> Wrap To Zero2/1
  Wrap To Zero2/1 -> Unit Delay3/1, NOT6/1
  NOT6/1 -> AND4/1
  Unit Delay3/1 -> Compare To Constant2/1, Sum1/2
  Compare To Constant2/1 -> AND4/2
  AND4/1 -> OR/1
  Data Type Conversion2/1 -> Sum1/1
  AND1/1 -> Data Type Conversion2/1

== system me375_robot/Count-to-speed (Single Pulse)/Triggered Subsystem1 ==
  Input : Inport
  Trigger : TriggerPort  VariantControl=(inherit)
  Constant1 : Constant
  Delay : Delay
  Delay1 : Delay  DelayLength=1
  Divide : Product  Inputs=*/
  Gain : Gain  Gain=1/3
  Minus : Sum  Inputs=+-
  Sum : Sum  Inputs=+++
  Unit Delay : UnitDelay  SampleTime=-1  HasFrameUpgradeWarning=on
  Out1 : Outport  InitialOutput=0
  Last round timestamp : Outport  Port=2
  wires:
  Input/1 -> Unit Delay/1, Minus/1
  Minus/1 -> Divide/2
  Constant1/1 -> Divide/1
  Divide/1 -> Sum/2, Delay/1, Delay1/1
  Unit Delay/1 -> Last round timestamp/1, Minus/2
  Delay/1 -> Sum/1
  Delay1/1 -> Sum/3
  Sum/1 -> Gain/1
  Gain/1 -> Out1/1

== system me375_robot/Enable//Reset/Subsystem ==
  Cool Down Signal : Inport
  function : TriggerPort  TriggerType=falling  VariantControl=(inherit)
  Abs : Abs  SaturateOnIntegerOverflow=off
  Constant : Constant
  Memory : Memory  InheritSampleTime=on
  OR : Logic  Operator=XOR  IconShape=distinctive  AllPortsSameDT=off  OutDataTypeStr=boolean
  Subtract : Sum  Inputs=+-
  Switch : Switch  Criteria=u2 > Threshold  Threshold=0.95  SaturateOnIntegerOverflow=off  InputSameDT=off
  Enable Out : Outport  InitialOutput=0
  wires:
  Switch/1 -> Memory/1, Enable Out/1
  Memory/1 -> Switch/3, OR/1
  Abs/1 -> Switch/2
  Subtract/1 -> Abs/1
  Constant/1 -> OR/2
  Cool Down Signal/1 -> Subtract/2
  OR/1 -> Switch/1, Subtract/1

== system me375_robot/Encoder Duo(non-Quadrature)/Function-Call Subsystem ==
  note: Accumulating
  note: Telling the direction by comparing pin states
  note: The other pin
  note: The other pin
  function : TriggerPort  TriggerType=function-call  VariantControl=(inherit)
  Constant1 : Constant
  Constant2 : Constant  Value=-1
  Constant4 : Constant
  Digital Input1 : arduinolib/Digital Input  pinNumber=pin_non_intr_1  mode=Input Pullup  Direction=input  SampleTime=-1  blockPlatform=arduino
  Sum : Sum  Inputs=|++
  Switch : Switch  Criteria=u2 > Threshold  SaturateOnIntegerOverflow=off  InputSameDT=off
  Unit Delay : UnitDelay  SampleTime=-1  HasFrameUpgradeWarning=on
  XOR : Logic  Operator=XOR  IconShape=distinctive  AllPortsSameDT=off  OutDataTypeStr=boolean
  enc on 2 : Outport  InitialOutput=0
  wires:
  Sum/1 -> Unit Delay/1, enc on 2/1
  Unit Delay/1 -> Sum/2
  Constant2/1 -> Switch/3
  Constant1/1 -> Switch/1
  XOR/1 -> Switch/2
  Switch/1 -> Sum/1
  Constant4/1 -> XOR/1
  Digital Input1/1 -> XOR/2

== system me375_robot/Encoder Duo(non-Quadrature)/Function-Call Subsystem1 ==
  note: Accumulating
  note: Telling the direction by comparing pin states
  note: The other pin
  note: The other pin
  function : TriggerPort  TriggerType=function-call  VariantControl=(inherit)
  Constant1 : Constant
  Constant2 : Constant  Value=-1
  Constant4 : Constant
  Digital Input1 : arduinolib/Digital Input  pinNumber=pin_non_intr_2  mode=Input Pullup  Direction=input  SampleTime=-1  blockPlatform=arduino
  Sum : Sum  Inputs=|++
  Switch : Switch  Criteria=u2 > Threshold  SaturateOnIntegerOverflow=off  InputSameDT=off
  Unit Delay : UnitDelay  SampleTime=-1  HasFrameUpgradeWarning=on
  XOR : Logic  Operator=XOR  IconShape=distinctive  AllPortsSameDT=off  OutDataTypeStr=boolean
  enc on 2 : Outport  InitialOutput=0
  wires:
  Sum/1 -> Unit Delay/1, enc on 2/1
  Unit Delay/1 -> Sum/2
  Constant2/1 -> Switch/3
  Constant1/1 -> Switch/1
  XOR/1 -> Switch/2
  Switch/1 -> Sum/1
  Constant4/1 -> XOR/1
  Digital Input1/1 -> XOR/2

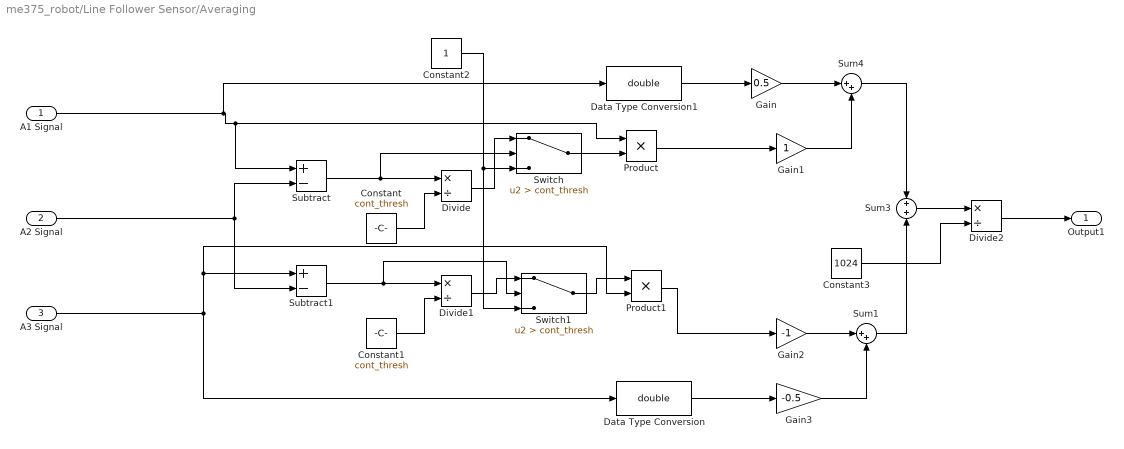
== system me375_robot/Line Follower Sensor/Averaging ==
  A1 Signal : Inport
  A2 Signal : Inport  Port=2
  A3 Signal : Inport  Port=3
  Constant : Constant  Value=cont_thresh
  Constant1 : Constant  Value=cont_thresh
  Constant2 : Constant
  Constant3 : Constant  Value=1024
  Data Type Conversion : DataTypeConversion  OutDataTypeStr=double  SaturateOnIntegerOverflow=off  RndMeth=Floor
  Data Type Conversion1 : DataTypeConversion  OutDataTypeStr=double  SaturateOnIntegerOverflow=off  RndMeth=Floor
  Divide : Product  Inputs=*/
  Divide1 : Product  Inputs=*/
  Divide2 : Product  Inputs=*/
  Gain : Gain  Gain=0.5
  Gain1 : Gain
  Gain2 : Gain  Gain=-1
  Gain3 : Gain  Gain=-0.5
  Product : Product
  Product1 : Product
  Subtract : Sum  Inputs=+-  OutDataTypeStr=int32
  Subtract1 : Sum  Inputs=+-  OutDataTypeStr=int32
  Sum1 : Sum  Inputs=|++
  Sum3 : Sum  Inputs=+|+
  Sum4 : Sum  Inputs=|++
  Switch : Switch  Criteria=u2 > Threshold  Threshold=cont_thresh  SaturateOnIntegerOverflow=off  InputSameDT=off
  Switch1 : Switch  Criteria=u2 > Threshold  Threshold=cont_thresh  SaturateOnIntegerOverflow=off  InputSameDT=off
  Output1 : Outport
  wires:
  A1 Signal/1 -> Data Type Conversion1/1, Product/1, Subtract/1
  A2 Signal/1 -> Subtract1/2, Subtract/2
  A3 Signal/1 -> Product1/2, Subtract1/1, Data Type Conversion/1
  Subtract/1 -> Switch/2, Divide/1
  Constant/1 -> Divide/2
  Constant1/1 -> Divide1/2
  Subtract1/1 -> Switch1/2, Divide1/1
  Switch/1 -> Product/2
  Switch1/1 -> Product1/1
  Product1/1 -> Gain2/1
  Divide/1 -> Switch/1
  Constant2/1 -> Switch1/3, Switch/3
  Divide1/1 -> Switch1/1
  Product/1 -> Gain1/1
  Gain/1 -> Sum4/1
  Gain1/1 -> Sum4/2
  Gain2/1 -> Sum1/1
  Gain3/1 -> Sum1/2
  Sum1/1 -> Sum3/2
  Sum4/1 -> Sum3/1
  Data Type Conversion/1 -> Gain3/1
  Data Type Conversion1/1 -> Gain/1
  Sum3/1 -> Divide2/1
  Constant3/1 -> Divide2/2
  Divide2/1 -> Output1/1

== system me375_robot/Motors Interface/Ctrl to Mtr Cmd (Braking) ==
  Ctrl Signal in : Inport
  Abs : Abs  SaturateOnIntegerOverflow=off
  Constant : Constant
  Gain : Gain  Gain=255
  Gain1 : Gain  Gain=255
  Saturation : Saturate  UpperLimit=1  LowerLimit=-1
  Sum : Sum  Inputs=|+-
  Switch : Switch  Criteria=u2 > Threshold  SaturateOnIntegerOverflow=off  InputSameDT=off
  Switch1 : Switch  Criteria=u2 > Threshold  SaturateOnIntegerOverflow=off  InputSameDT=off
  PWM Out 1 : Outport
  PWM Out 2 : Outport  Port=2
  wires:
  Gain1/1 -> PWM Out 2/1
  Gain/1 -> PWM Out 1/1
  Switch/1 -> Gain/1
  Switch1/1 -> Gain1/1
  Sum/1 -> Switch/3, Switch1/1
  Abs/1 -> Sum/2
  Ctrl Signal in/1 -> Saturation/1
  Saturation/1 -> Switch/2, Switch1/2, Abs/1
  Constant/1 -> Switch/1, Switch1/3, Sum/1

== system me375_robot/Motors Interface/Ctrl to Mtr Cmd (Braking)1 ==
  Ctrl Signal in : Inport
  Abs : Abs  SaturateOnIntegerOverflow=off
  Constant : Constant
  Gain : Gain  Gain=255
  Gain1 : Gain  Gain=255
  Saturation : Saturate  UpperLimit=1  LowerLimit=-1
  Sum : Sum  Inputs=|+-
  Switch : Switch  Criteria=u2 > Threshold  SaturateOnIntegerOverflow=off  InputSameDT=off
  Switch1 : Switch  Criteria=u2 > Threshold  SaturateOnIntegerOverflow=off  InputSameDT=off
  PWM Out 1 : Outport
  PWM Out 2 : Outport  Port=2
  wires:
  Gain1/1 -> PWM Out 2/1
  Gain/1 -> PWM Out 1/1
  Switch/1 -> Gain/1
  Switch1/1 -> Gain1/1
  Sum/1 -> Switch/3, Switch1/1
  Abs/1 -> Sum/2
  Ctrl Signal in/1 -> Saturation/1
  Saturation/1 -> Switch/2, Switch1/2, Abs/1
  Constant/1 -> Switch/1, Switch1/3, Sum/1

== system me375_robot/Count-to-Speed/Stop Detection/Triggered Subsystem2 ==
  Trigger : TriggerPort  VariantControl=(inherit)
  Constant3 : Constant
  Unit Delay : UnitDelay  SampleTime=-1  HasFrameUpgradeWarning=on
  XOR : Logic  Operator=XOR  IconShape=distinctive  AllPortsSameDT=off  OutDataTypeStr=boolean
  Out1 : Outport  InitialOutput=0
  wires:
  Constant3/1 -> XOR/2
  Unit Delay/1 -> XOR/1
  XOR/1 -> Out1/1, Unit Delay/1

== system me375_robot/Count-to-Speed (Full Rotation)/Stop Detection/Triggered Subsystem2 ==
  Trigger : TriggerPort  VariantControl=(inherit)
  Constant3 : Constant
  Unit Delay : UnitDelay  SampleTime=-1  HasFrameUpgradeWarning=on
  XOR : Logic  Operator=XOR  IconShape=distinctive  AllPortsSameDT=off  OutDataTypeStr=boolean
  Out1 : Outport  InitialOutput=0
  wires:
  XOR/1 -> Unit Delay/1, Out1/1
  Unit Delay/1 -> XOR/1
  Constant3/1 -> XOR/2

== system me375_robot/Count-to-speed (Single Pulse)/Stop Detection/Triggered Subsystem2 ==
  Trigger : TriggerPort  VariantControl=(inherit)
  Constant3 : Constant
  Unit Delay : UnitDelay  SampleTime=-1  HasFrameUpgradeWarning=on
  XOR : Logic  Operator=XOR  IconShape=distinctive  AllPortsSameDT=off  OutDataTypeStr=boolean
  Out1 : Outport  InitialOutput=0
  wires:
  XOR/1 -> Unit Delay/1, Out1/1
  Unit Delay/1 -> XOR/1
  Constant3/1 -> XOR/2

== matlab function me375_robot/MATLAB Function ==
function y()
a = arduino();
configurePin(a,'D18','pullup');
configurePin(a,'D19','pullup');
configurePin(a,'D2','pullup');
configurePin(a,'D3','pullup');
